simulink model "model"  (R2023a)
settings: Solver=VariableStepAuto  StartTime=0.0  StopTime=1000  RelTol=1e-3
InitFcn:
  | init
undefined symbols (not defined in the file): g, k, Kd, Ki, Kp, M1, M2, mu
settings Model: Creator=Zonularity  LastModifiedBy=Zonularity

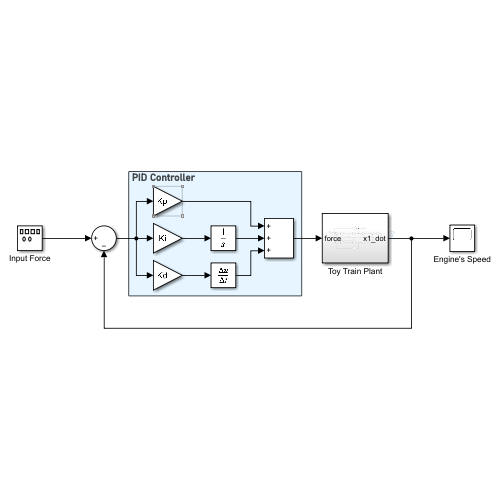
[thumbnail: Simulink's stored preview of the top-level diagram]
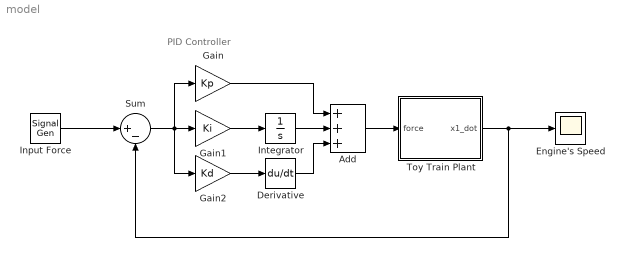
== system model ==
  note: PID Controller
  Add : Sum  Inputs=+++
  Derivative : Derivative
  Engine's Speed : Scope
  Gain : Gain  Gain=Kp
  Gain1 : Gain  Gain=Ki
  Gain2 : Gain  Gain=Kd
  Input Force : SignalGenerator  WaveForm=square  Amplitude=-1  Frequency=0.001
  Integrator : Integrator
  Sum : Sum  Inputs=|+-
  Toy Train Plant : Subsystem
  wires:
  Toy Train Plant/1(x1_dot) -> Sum/2, Engine's Speed/1
  Input Force/1 -> Sum/1
  Gain1/1 -> Integrator/1
  Gain2/1 -> Derivative/1
  Integrator/1 -> Add/2
  Derivative/1 -> Add/3
  Gain/1 -> Add/1
  Sum/1 -> Gain2/1, Gain/1, Gain1/1
  Add/1 -> Toy Train Plant/1(force)

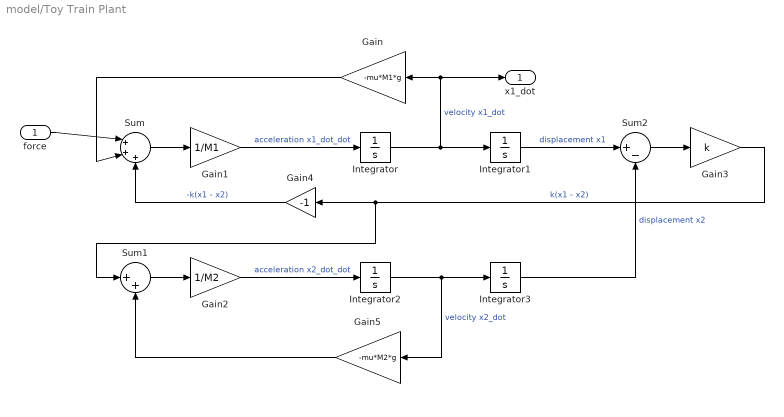
== system model/Toy Train Plant ==
  force : Inport
  Gain : Gain  Gain=-mu*M1*g
  Gain1 : Gain  Gain=1/M1
  Gain2 : Gain  Gain=1/M2
  Gain3 : Gain  Gain=k
  Gain4 : Gain  Gain=-1
  Gain5 : Gain  Gain=-mu*M2*g
  Integrator{,1..3} (4 alike) : Integrator
  Sum : Sum  Inputs=|+++
  Sum1 : Sum  Inputs=|++
  Sum2 : Sum  Inputs=|+-
  x1_dot : Outport
  wires:
  Gain4/1 -> Sum/3  "-k(x1 - x2)"
  Gain3/1 -> Sum1/1, Gain4/1  "k(x1 - x2)"
  Integrator2/1 -> Gain5/1, Integrator3/1  "velocity x2_dot"
  Integrator/1 -> Integrator1/1, x1_dot/1, Gain/1  "velocity x1_dot"
  Gain2/1 -> Integrator2/1  "acceleration x2_dot_dot"
  Gain5/1 -> Sum1/2
  Integrator1/1 -> Sum2/1  "displacement x1"
  Sum2/1 -> Gain3/1
  Gain1/1 -> Integrator/1  "acceleration x1_dot_dot"
  Sum/1 -> Gain1/1
  Sum1/1 -> Gain2/1
  Integrator3/1 -> Sum2/2  "displacement x2"
  Gain/1 -> Sum/2
  force/1 -> Sum/1
